simulink model "Arduino_MotorControl2024"  (R2024a)
settings: Solver=FixedStepDiscrete  StartTime=0.0  StopTime=10.0  FixedStep=0.05  RelTol=1e-3  EnableMultiTasking=on
libraries: arduinolib x7
settings Model: ExtModeTrigDuration=2  Creator=Tasneem  LastModifiedBy=Tasneem
settings SolverCC: AutoInsertRateTranBlk=on
settings OptimizationCC: EnhancedBackFolding=on  PassReuseOutputArgsAs=Individual arguments  ZeroExternalMemoryAtStartup=off  ZeroInternalMemoryAtStartup=off  MaxStackSize=64  OptimizeBlockOrder=speed  DifferentSizesBufferReuse=on  OptimizationCustomize=off  EfficientTunableParamExpr=on
settings DebuggingCC: ParameterTunabilityLossMsg=error
settings HardwareCC: ProdBitPerInt=16  ProdBitPerPointer=16  ProdBitPerSizeT=16  ProdBitPerPtrDiffT=16  ProdLargestAtomicFloat=None  ProdWordSize=8  ProdHWDeviceType=Atmel->AVR
settings SFSimCC: MATLABDynamicMemAlloc=off
settings RTWCC: Description=Embedded Coder  SystemTargetFile=ert.tlc  HardwareBoard=Arduino Uno  TemplateMakefile=ert_default_tmf  Toolchain=Arduino AVR  BuildConfiguration=Faster Runs
settings CodeAppCC: ForceParamTrailComments=on  IgnoreCustomStorageClasses=off  OperatorAnnotations=on  SimulinkDataObjDesc=on  SFDataObjDesc=on  InsertBlockDesc=on
settings ERTTargetCC: SupportContinuousTime=on  SupportVariableSizeSignals=on  ExtModeTransport=3  ExtModeStaticAlloc=on  ExtModeAutomaticAllocSize=off  ExtModeStaticAllocSize=250  ExtModeMexFile=ext_xcp  ExtModeIntrfLevel=Level2 - Open
settings ConfigComp: CovBoundaryAbsTol=1.0e-5

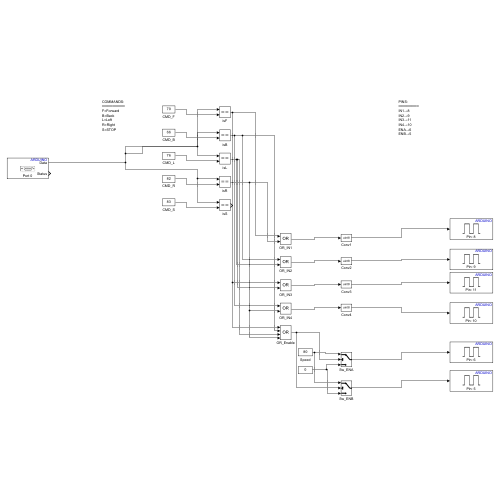
[thumbnail: Simulink's stored preview of the top-level diagram]
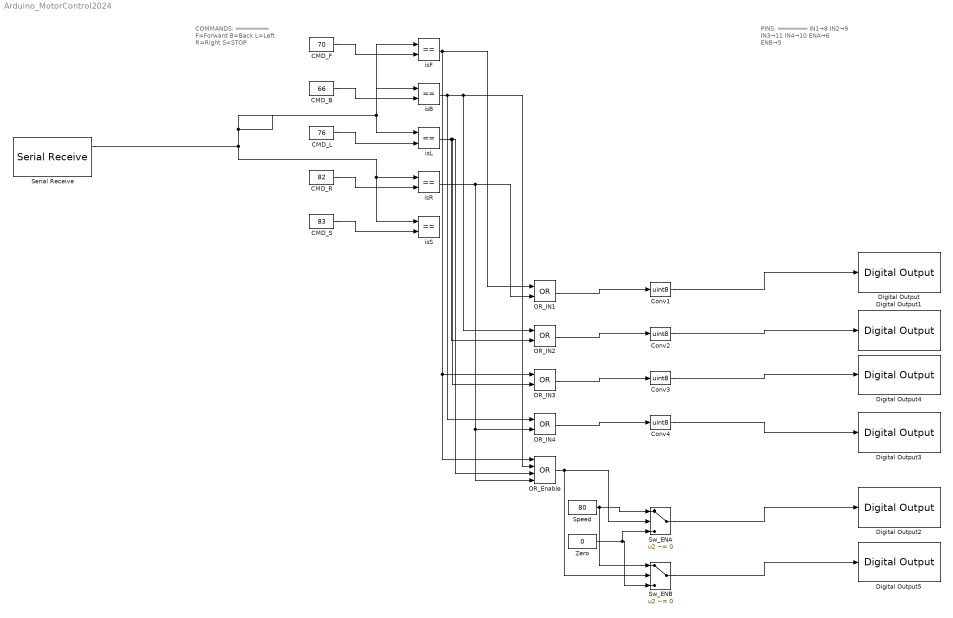
== system Arduino_MotorControl2024 ==
  note: PINS:
      | ════════
      | IN1→8
      | IN2→9
      | IN3→11
      | IN4→10
      | ENA→6
      | ENB→5
  note: COMMANDS:
      | ═════════
      | F=Forward
      | B=Back
      | L=Left
      | R=Right
      | S=STOP
  CMD_B : Constant  Value=66  OutDataTypeStr=uint8
  CMD_F : Constant  Value=70  OutDataTypeStr=uint8
  CMD_L : Constant  Value=76  OutDataTypeStr=uint8
  CMD_R : Constant  Value=82  OutDataTypeStr=uint8
  CMD_S : Constant  Value=83  OutDataTypeStr=uint8
  Conv{1..4} (4 alike) : DataTypeConversion  OutDataTypeStr=uint8  SaturateOnIntegerOverflow=off  RndMeth=Floor
  Digital Output : arduinolib/Digital Output  pinNumber=8  Direction=output  blockPlatform=arduino
  Digital Output1 : arduinolib/Digital Output  pinNumber=9  Direction=output  blockPlatform=arduino
  Digital Output2 : arduinolib/Digital Output  pinNumber=6  Direction=output  blockPlatform=arduino
  Digital Output3 : arduinolib/Digital Output  pinNumber=10  Direction=output  blockPlatform=arduino
  Digital Output4 : arduinolib/Digital Output  pinNumber=11  Direction=output  blockPlatform=arduino
  Digital Output5 : arduinolib/Digital Output  pinNumber=5  Direction=output  blockPlatform=arduino
  OR_Enable : Logic  Operator=OR  Inputs=4  AllPortsSameDT=off  OutDataTypeStr=boolean
  OR_IN{1..4} (4 alike) : Logic  Operator=OR  AllPortsSameDT=off  OutDataTypeStr=boolean
  Serial Receive : arduinolib/Serial Receive  portNumber=0  DataType=uint8  blockPlatform=ARDUINO  TimeOut=0  MaxDataLength=10  isARMArch=off  DataLengthOption=Length via dialog  Datalength=1  Header=[]  Terminator=[]  SampleTime=0.1  ShowOutStatus=on
  Speed : Constant  Value=80  OutDataTypeStr=uint8
  Sw_ENA : Switch  Criteria=u2 ~= 0  SaturateOnIntegerOverflow=off  InputSameDT=off
  Sw_ENB : Switch  Criteria=u2 ~= 0  SaturateOnIntegerOverflow=off  InputSameDT=off
  Zero : Constant  Value=0  OutDataTypeStr=uint8
  isB : RelationalOperator  Operator===  OutDataTypeStr=boolean  RndMeth=Simplest  InputSameDT=off
  isF : RelationalOperator  Operator===  OutDataTypeStr=boolean  RndMeth=Simplest  InputSameDT=off
  isL : RelationalOperator  Operator===  OutDataTypeStr=boolean  RndMeth=Simplest  InputSameDT=off
  isR : RelationalOperator  Operator===  OutDataTypeStr=boolean  RndMeth=Simplest  InputSameDT=off
  isS : RelationalOperator  Operator===  OutDataTypeStr=boolean  RndMeth=Simplest  InputSameDT=off
  wires:
  Serial Receive/1 -> isB/1, isL/1, isF/1, isR/1, isS/1
  CMD_F/1 -> isF/2
  CMD_B/1 -> isB/2
  CMD_L/1 -> isL/2
  CMD_R/1 -> isR/2
  CMD_S/1 -> isS/2
  isF/1 -> OR_IN3/1, OR_Enable/1, OR_IN1/1
  isR/1 -> OR_Enable/4, OR_IN4/2, OR_IN1/2
  isB/1 -> OR_Enable/2, OR_IN2/1, OR_IN4/1
  isL/1 -> OR_Enable/3, OR_IN3/2, OR_IN2/2
  OR_IN1/1 -> Conv1/1
  OR_IN2/1 -> Conv2/1
  OR_IN3/1 -> Conv3/1
  OR_IN4/1 -> Conv4/1
  Speed/1 -> Sw_ENA/1, Sw_ENB/1
  OR_Enable/1 -> Sw_ENA/2, Sw_ENB/2
  Zero/1 -> Sw_ENA/3, Sw_ENB/3
  Conv1/1 -> Digital Output/1
  Conv2/1 -> Digital Output1/1
  Conv3/1 -> Digital Output4/1
  Conv4/1 -> Digital Output3/1
  Sw_ENA/1 -> Digital Output2/1
  Sw_ENB/1 -> Digital Output5/1
